simulink model "bustest"  (R2018a)
settings: Solver=VariableStepAuto  StartTime=0.0  StopTime=10.0  RelTol=1e-3
undefined symbols (not defined in the file or in its folder): BaseVoltage, ControlModes, ILDC, m, n, RCReg1, Reg1i, Reg1v, TReg1
(part 1 of 2)
settings Model: Creator=Michael Girbino  LastModifiedBy=Michael Girbino
settings CodeAppCC: StateflowObjectComments=on

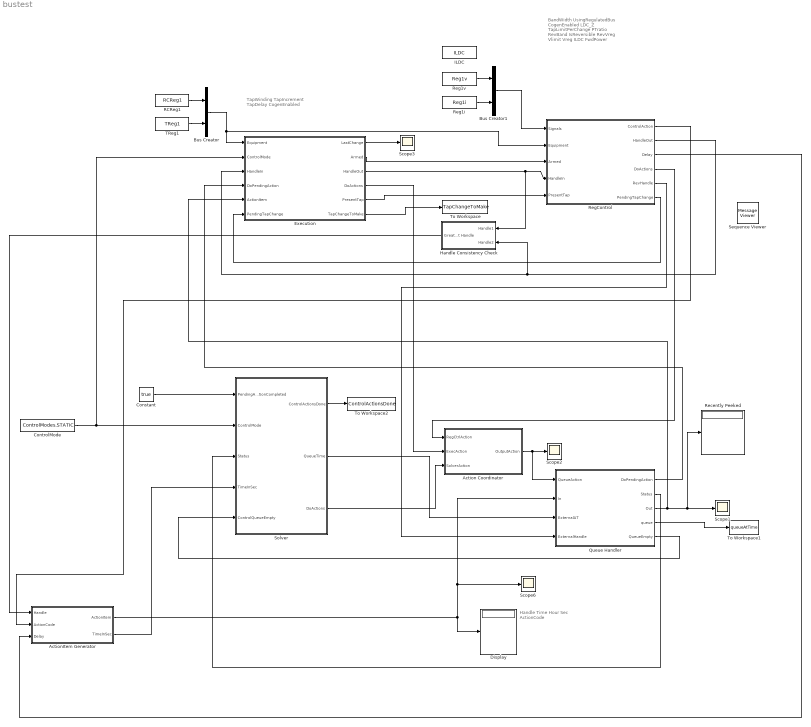
== system bustest ==
  note: BandWidth
      | UsingRegulatedBus
      | CogenEnabled
      | LDC_Z
      | TapLimitPerChange
      | PTratio
      | RevBand
      | IsReversible
      | RevVreg
      | Vlimit
      | Vreg
      | ILDC
      | FwdPower
  note: Handle
      | Time
      | Hour
      | Sec
      | ActionCode
  note: TapWinding
      | TapIncrement
      | TapDelay
      | CogenEnabled
  Action Coordinator : Stateflow chart  TreatAsAtomicUnit=on
  ActionItem Generator : Subsystem
  Bus Creator : BusCreator  Inputs=2  OutDataTypeStr=Bus: EquipmentBus
  Bus Creator1 : BusCreator  Inputs=2  OutDataTypeStr=Bus: SignalBus
  Constant : Constant  Value=true  OutDataTypeStr=boolean
  ControlMode : Constant  Value=ControlModes.STATIC  OutDataTypeStr=Enum: ControlModes
  Display : Display
  Execution : Stateflow chart  TreatAsAtomicUnit=on
  Handle Consistency Check : Subsystem
  ILDC : Constant  Value=ILDC
  Queue Handler : Stateflow chart  TreatAsAtomicUnit=on
  RCReg1 : Constant  Value=RCReg1
  Recently Peeked : Display
  Reg1i : Constant  Value=Reg1i
  Reg1v : Constant  Value=Reg1v
  RegControl : Stateflow chart  TreatAsAtomicUnit=on
  Scope{1..3,6} (4 alike) : Scope
  Sequence Viewer : MessageViewer
  Solver : Stateflow chart  TreatAsAtomicUnit=on
  TReg1 : Constant  Value=TReg1
  To Workspace : ToWorkspace  VariableName=TapChangeToMake  SaveFormat=Timeseries  SampleTime=-1
  To Workspace1 : ToWorkspace  VariableName=queueAtTime  SaveFormat=Structure With Time  SampleTime=-1
  To Workspace2 : ToWorkspace  VariableName=ControlActionsDone  SaveFormat=Timeseries  SampleTime=-1
  wires:
  Queue Handler/5(QueueEmpty) -> Solver/5(ControlQueueEmpty)
  Queue Handler/4(queue) -> To Workspace1/1
  Constant/1 -> Solver/1(PendingActionCompleted)
  ActionItem Generator/2(TimeInSec) -> Solver/4(TimeInSec)
  Queue Handler/2(Status) -> Solver/3(Status)
  ControlMode/1 -> Execution/2(ControlMode), Solver/2(ControlMode)
  Solver/2(QueueTime) -> Queue Handler/3(ExternalAT)
  Queue Handler/3(Out) -> Recently Peeked/1, Scope1/1, Execution/5(ActionItem)
  ActionItem Generator/1(ActionItem) -> Scope6/1, Queue Handler/2(In), Display/1
  Solver/1(ControlActionsDone) -> To Workspace2/1
  RegControl/1(ControlAction) -> ActionItem Generator/2(ActionCode)
  Action Coordinator/1(OutputAction) -> Queue Handler/1(QueueAction), Scope2/1
  Solver/3(DoActions) -> Action Coordinator/3(SolverAction)
  Execution/4(DoActions) -> Action Coordinator/2(ExecAction)
  RegControl/4(DoActions) -> Action Coordinator/1(RegCtrlAction)
  RegControl/3(Delay) -> ActionItem Generator/3(Delay)
  RegControl/2(HandleOut) -> Handle Consistency Check/2(Handle2), Execution/3(HandleIn)
  RegControl/5(RevHandle) -> Queue Handler/4(ExternalHandle)
  Execution/3(HandleOut) -> Handle Consistency Check/1(Handle1), RegControl/4(HandleIn)
  Execution/2(Armed) -> RegControl/3(Armed)
  Queue Handler/1(DoPendingAction) -> Execution/4(DoPendingAction)
  Execution/6(TapChangeToMake) -> To Workspace/1
  RegControl/6(PendingTapChange) -> Execution/6(PendingTapChange)
  Execution/1(LastChange) -> Scope3/1
  Handle Consistency Check/1(Greatest Handle) -> ActionItem Generator/1(Handle)
  Execution/5(PresentTap) -> RegControl/5(PresentTap)
  RCReg1/1 -> Bus Creator/1
  TReg1/1 -> Bus Creator/2
  Reg1v/1 -> Bus Creator1/1
  Reg1i/1 -> Bus Creator1/2
  Bus Creator/1 -> RegControl/2(Equipment), Execution/1(Equipment)
  Bus Creator1/1 -> RegControl/1(Signals)

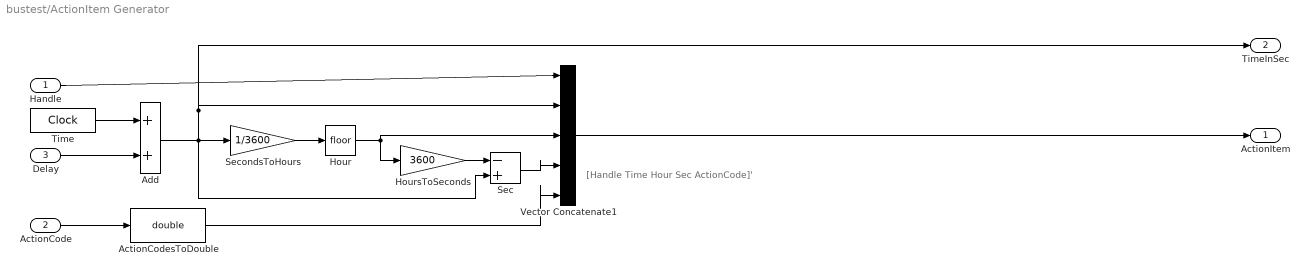
== system bustest/ActionItem Generator ==
  note: [Handle Time Hour Sec ActionCode]'
  Handle : Inport
  ActionCode : Inport  Port=2
  Delay : Inport  Port=3
  ActionCodesToDouble : DataTypeConversion  OutDataTypeStr=double
  Add : Sum
  Hour : Rounding
  HoursToSeconds : Gain  Gain=3600
  Sec : Sum  Inputs=-+
  SecondsToHours : Gain  Gain=1/3600
  Time : DigitalClock
  Vector Concatenate1 : Concatenate  NumInputs=5
  ActionItem : Outport
  TimeInSec : Outport  Port=2
  wires:
  Add/1 -> Sec/2, SecondsToHours/1, TimeInSec/1, Vector Concatenate1/2
  Hour/1 -> Vector Concatenate1/3, HoursToSeconds/1
  SecondsToHours/1 -> Hour/1
  Vector Concatenate1/1 -> ActionItem/1
  HoursToSeconds/1 -> Sec/1
  Handle/1 -> Vector Concatenate1/1
  Sec/1 -> Vector Concatenate1/4
  Delay/1 -> Add/2
  Time/1 -> Add/1
  ActionCode/1 -> ActionCodesToDouble/1
  ActionCodesToDouble/1 -> Vector Concatenate1/5

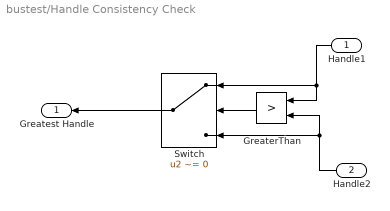
== system bustest/Handle Consistency Check ==
  Handle1 : Inport
  Handle2 : Inport  Port=2
  GreaterThan : RelationalOperator  Operator=>  RndMeth=Simplest
  Switch : Switch  Criteria=u2 ~= 0
  Greatest Handle : Outport
  wires:
  Handle2/1 -> GreaterThan/2, Switch/3
  GreaterThan/1 -> Switch/2
  Handle1/1 -> GreaterThan/1, Switch/1
  Switch/1 -> Greatest Handle/1

== stateflow chart bustest/Execution ==
  settings: executeAtInitialization=1
  state Push(CodeVal, DelayVal) [function]
    (default) -> (junction 341) : {ActionCode = CodeVal;
        | Delay = DelayVal;
        | HandleOut = HandleOut + 1;
        | DoActions.data = QueueActions.PUSH;
        | send(DoActions);}
  state ControlFlow
    state MakingTapChange
      state StaticTapChange
        (default) -> (junction 165) : {TapChangeToMake = AtLeastOneTap(PendingTapChange, TapIncrement(TapWinding));
            | % reset to no change = change - 1 program will determin if another is needed:
            | PendingTapChange = 0;
            | Armed = false;}
      state EventDrivenTapChange
        (default) -> (junction 189) : {[TapChangeToMake LocalPendingTapChange] =...
            |  OneInDirectionOf(LocalPendingTapChange, TapIncrement(TapWinding));
            | PresentTap(TapWinding) = PresentTap(TapWinding) + TapChangeToMake;}
        (junction 189) -> (junction 190) [order 1] : [PendingTapChange ~= 0]
        (junction 189) -> (junction 191) [order 2] : {Armed = false;}
        (junction 190) -> (junction 192) : {Push(ActionCodes.ACTION_TAPCHANGE, TapDelay);}
        (junction 192) -> (junction 191)
      state TimeDrivenTapChange
        (default) -> (junction 200) : {[TapChangeToMake LocalPendingTapChange] =...
            |  OneInDirectionOf(LocalPendingTapChange, TapIncrement(TapWinding));
            | PresentTap(TapWinding) = PresentTap(TapWinding) + TapChangeToMake;}
        (junction 200) -> (junction 202) [order 1] : [PendingTapChange ~= 0]
        (junction 200) -> (junction 203) [order 2] : {Armed = false;}
        (junction 202) -> (junction 201) : {Push(ActionCodes.ACTION_TAPCHANGE, TapDelay);}
        (junction 201) -> (junction 203)
      state MultiRateTapChange
        (default) -> (junction 210) : {[TapChangeToMake, LocalPendingTapChange] =...
            |  OneInDirectionOf(LocalPendingTapChange, TapIncrement(TapWinding));
            | PresentTap(TapWinding) = PresentTap(TapWinding) + TapChangeToMake;}
        (junction 210) -> (junction 212) [order 1] : [PendingTapChange ~= 0]
        (junction 210) -> (junction 213) [order 2] : {Armed = false;}
        (junction 212) -> (junction 211) : {Push(ActionCodes.ACTION_TAPCHANGE, TapDelay);}
        (junction 211) -> (junction 213)
      state Finished
        en: EXIT_TAPCHANGE = true;
      (default) -> (junction 132)
      (junction 132) -> (junction 133) [order 1] : % Check to make sure control has not reset:
          | [PendingTapChange == 0]
      (junction 132) -> (junction 163) [order 2]
      (junction 133) -> (junction 135) : {Armed = false;}
      (junction 163) -> StaticTapChange [order 1] : [ControlMode == ControlModes.STATIC]
      (junction 163) -> (junction 167) [order 2]
      StaticTapChange -> (junction 170)
      (junction 167) -> EventDrivenTapChange [order 1] : [ControlMode == ControlModes.EVENTDRIVEN]
      (junction 167) -> (junction 171) [order 2]
      EventDrivenTapChange -> (junction 169)
      (junction 169) -> (junction 170)
      (junction 170) -> (junction 174)
      (junction 171) -> TimeDrivenTapChange [order 1] : [ControlMode == ControlModes.TIMEDRIVEN]
      (junction 171) -> (junction 175) [order 2]
      TimeDrivenTapChange -> (junction 173)
      (junction 173) -> (junction 174)
      (junction 174) -> (junction 178)
      (junction 175) -> MultiRateTapChange [order 1] : [ControlMode == ControlModes.MULTIRATE]
      (junction 175) -> (junction 179) [order 2]
      (junction 178) -> (junction 180)
      MultiRateTapChange -> (junction 357)
      (junction 357) -> (junction 179)
      (junction 180) -> (junction 357)
      (junction 179) -> ControlFlow.MakingTapChange.Finished
      (junction 135) -> ControlFlow.MakingTapChange.Finished
    state Reversing
      state FlipCogen
        (default) -> (junction 252)
        (junction 252) -> (junction 253) [order 1] : [InCogenMode]
        (junction 252) -> (junction 254) [order 2] : {InCogenMode = true;}
        (junction 253) -> (junction 255) : {InCogenMode = false;}
        (junction 255) -> (junction 254)
      state FlipReverse
        (default) -> (junction 263)
        (junction 263) -> (junction 264) [order 1] : [InReverseMode]
        (junction 263) -> (junction 265) [order 2] : {InReverseMode = true;}
        (junction 264) -> (junction 266) : {InReverseMode = false;}
        (junction 266) -> (junction 265)
      state Finished
        en: EXIT_REVERSE = true;
      (default) -> (junction 229)
      (junction 229) -> (junction 230) [order 1] : [ReversePending]
      (junction 229) -> (junction 231) [order 2]
      (junction 230) -> (junction 242)
      (junction 242) -> (junction 238) [order 1] : [CogenEnabled]
      (junction 242) -> FlipReverse [order 2]
      (junction 238) -> FlipCogen : % Cogen mode takes precedence if present
      FlipCogen -> (junction 245)
      FlipReverse -> (junction 240)
      (junction 245) -> (junction 240)
      (junction 240) -> (junction 232) : {ReversePending = false;}
      (junction 232) -> (junction 231)
      (junction 231) -> ControlFlow.Reversing.Finished
    state Finished
    (default) -> (junction 115) : {AssignInputsToLocals();
        | ResetTransitionFlags();}
    (junction 115) -> MakingTapChange [order 1] : [Code == ActionCodes.ACTION_TAPCHANGE]
    (junction 115) -> (junction 119) [order 2]
    MakingTapChange -> (junction 117) : [EXIT_TAPCHANGE]
    (junction 117) -> (junction 118)
    (junction 118) -> (junction 122)
    (junction 119) -> Reversing [order 1] : [Code == ActionCodes.ACTION_REVERSE]
    (junction 119) -> (junction 123) [order 2]
    Reversing -> (junction 122)
    (junction 122) -> (junction 124) : [EXIT_REVERSE]
    (junction 124) -> (junction 123)
    (junction 123) -> ControlFlow.Finished
  state AssignInputsToLocals [function]
    note: TapWinding
        | TapIncrement
        | TapDelay
        | CogenEnabled
    (default) -> (junction 365) : {% From Script:
        | TapWinding = Equipment.RCReg1.xsfWinding;
        | TapIncrement = Equipment.TReg1.Winding(TapWinding).TapIncrement;
        | TapDelay = Equipment.RCReg1.TapDelay;
        | CogenEnabled = Equipment.RCReg1.CogenEnabled;
        | % From the ControlQueue:
        | Code = ...
        | ActionItem(NewControlQueueFields.ActionCode);
        | % PendingTapChange:
        | LocalPendingTapChange = PendingTapChange;}
    (junction 365) -> (junction 372) [order 1] : [HandleIn > HandleOut]
    (junction 365) -> (junction 373) [order 2]
    (junction 372) -> (junction 374) : {HandleOut = HandleIn;}
    (junction 374) -> (junction 373)
    (junction 373) -> (junction 375)
  state ChangeToMake = AtLeastOneTap(ProposedChange, Increment) [function]
    note: Called in STATIC mode
        | Changes 70% of the way but at least one tap, subject to maximum allowable tap change
    (default) -> (junction 283) : {NumTaps = floor(0.7 * abs(ProposedChange)/Increment);}
    (junction 283) -> (junction 284) [order 1] : [NumTaps == 0]
    (junction 283) -> (junction 285) [order 2]
    (junction 284) -> (junction 286) : {NumTaps = 1;} % At least 1 tap
    (junction 286) -> (junction 285)
    (junction 285) -> (junction 293)
    (junction 293) -> (junction 290) [order 1] : [NumTaps > TapLimitPerChange]
    (junction 293) -> (junction 294) [order 2]
    (junction 290) -> (junction 295) : {NumTaps = TapLimitPerChange;} % Bound by maximum
    (junction 295) -> (junction 294)
    (junction 294) -> (junction 302) : {LastChange = NumTaps;}
    (junction 302) -> (junction 303) [order 1] : % Check sign on change:
        | [ProposedChange > 0]
    (junction 302) -> (junction 304) [order 2] : {ChangeToMake = -1*NumTaps*Increment;
        | LastChange = -1*NumTaps;}
    (junction 303) -> (junction 305) : {ChangeToMake =...
        |  NumTaps*Increment;}
    (junction 305) -> (junction 304)
    (junction 304) -> (junction 306)
  state ResetTransitionFlags [function]
    (default) -> (junction 377) : {EXIT_TAPCHANGE = false;
        | EXIT_REVERSE = false;}
  state [ChangeToMake, NewProposedChange] = OneInDirectionOf(ProposedChange, Increment) [function]
    note: Computes the amount of one tap change in the direction of the pending tapchange
        | Automatically decrements the proposed change by that amount
    (default) -> (junction 318) : {LastChange = 0;}
    (junction 318) -> (junction 319) [order 1] : [ProposedChange > 0]
    (junction 318) -> (junction 320) [order 2] : {ChangeToMake = -1*Increment;
        | LastChange = -1;
        | NewProposedChange = ProposedChange + Increment;}
    (junction 319) -> (junction 321) : {ChangeToMake = Increment;
        | LastChange = 1;
        | NewProposedChange =...
        |  ProposedChange - Increment;}
    (junction 321) -> (junction 320)
    (junction 320) -> (junction 329)
    (junction 329) -> (junction 330) [order 1] : [abs(NewProposedChange) < 0.9*Increment]
    (junction 329) -> (junction 331) [order 2]
    (junction 330) -> (junction 332) : {NewProposedChange = 0;}
    (junction 332) -> (junction 331)
    (junction 331) -> (junction 333)
  (default) -> ControlFlow : DoPendingAction
  data: CodeVal function_input; DelayVal function_input; ProposedChange function_input; Increment function_input; ChangeToMake function_output; ProposedChange function_input; Increment function_input; ChangeToMake function_output; NewProposedChange function_output; Equipment input Bus: EquipmentBus; LastChange output double; Change local double; NumTaps local uint8; ControlMode input Enum: ControlModes; HandleIn input double; Armed output boolean; HandleOut output double =0; DoActions output boolean =false; PresentTap output double; EXIT_REVERSE local boolean; InReverseMode local boolean; EXIT_TAPCHANGE local boolean; ReversePending local boolean; InCogenMode local boolean; DoPendingAction input boolean; TapWinding local uint8; TapIncrement local double; TapDelay local double; CogenEnabled local boolean =false; Code local Enum: ActionCodes; ActionItem input double size=[1 5]; TapChangeToMake output double; PendingTapChange input double; LocalPendingTapChange local double

== stateflow chart bustest/Solver ==
  state ControlFlow
    note: Static
        | - placeholder QueueTime
        | - DoNearestActions
    note: Event-driven
        | - QueueTime is current time
        | - DoNearestActions
    note: Time-driven
        | - QueueTime is current time
        | - DoActions
    note: Multirate
        | - QueueTime is current time
        | - DoMultiRate
    (default) -> (junction 25)
    (junction 25) -> (junction 26) [order 1] : [ControlMode == ControlModes.STATIC]
    (junction 25) -> (junction 29) [order 2]
    (junction 26) -> (junction 54)
    (junction 54) -> (junction 55) [order 1] : [LocalControlQueueEmpty]
        | % execute nearest set of control actions, but leave time where it is
    (junction 54) -> (junction 56) [order 2] : {QueueTime = 0; %[0 0] xHour, xSec
        | DoActions.data = QueueActions.DO_NEAREST_ACTIONS;
        | send(DoActions);
        | % ignores time advancement
        | }
    (junction 55) -> (junction 57) : {ControlActionsDone = true;}
    (junction 57) -> (junction 56)
    (junction 56) -> (junction 27)
    (junction 27) -> (junction 28)
    (junction 28) -> (junction 32)
    (junction 29) -> (junction 30) [order 1] : [ControlMode == ControlModes.EVENTDRIVEN]
        | % execute nearest set of control actions and advance time to that time
    (junction 30) -> (junction 65) : {QueueTime = TimeInSec; %xHour, xSec
        | DoActions.data = QueueActions.DO_NEAREST_ACTIONS;
        | send(DoActions);}
    (junction 29) -> (junction 33) [order 2]
    (junction 65) -> (junction 66) [order 1] : [~PendingActionCompleted]
    (junction 65) -> (junction 67) [order 2]
    (junction 66) -> (junction 68) : {ControlActionsDone = true;
        | % advances time to the next event
        | }
    (junction 68) -> (junction 67)
    (junction 67) -> (junction 31)
    (junction 31) -> (junction 32)
    (junction 32) -> (junction 36)
    (junction 33) -> (junction 34) [order 1] : [ControlMode == ControlModes.TIMEDRIVEN]
        |  % Do all actions having and action time <= specified time
    (junction 33) -> (junction 37) [order 2]
    (junction 34) -> (junction 78) : {QueueTime = TimeInSec; %xHour, xSec
        | DoActions.data = QueueActions.DO_ACTIONS;
        | send(DoActions);}
    (junction 78) -> (junction 80) [order 1] : [~PendingActionCompleted]
    (junction 78) -> (junction 79) [order 2]
    (junction 80) -> (junction 82) : {ControlActionsDone = true;
        | }
    (junction 82) -> (junction 79)
    (junction 79) -> (junction 35)
    (junction 35) -> (junction 36)
    (junction 36) -> (junction 40)
    (junction 37) -> (junction 38) [order 1] : [ControlMode == ControlModes.MULTIRATE]
        |  % Execute the nearest set of control actions, but leave time where it is
    (junction 37) -> (junction 41) [order 2]
    (junction 38) -> (junction 91) : {QueueTime =TimeInSec; %xHour, xSec
        | DoActions.data = QueueActions.DO_MULTIRATE;
        | send(DoActions);}
    (junction 91) -> (junction 88) [order 1] : [~PendingActionCompleted]
    (junction 91) -> (junction 87) [order 2]
    (junction 88) -> (junction 92) : {ControlActionsDone = true;
        | }
    (junction 92) -> (junction 87)
    (junction 87) -> (junction 39)
    (junction 39) -> (junction 40)
    (junction 40) -> (junction 42)
    (junction 42) -> (junction 41)
    (junction 41) -> (junction 43)
  state QueueEmptyCase
    en: LocalControlQueueEmpty = true;
  (default) -> ControlFlow
  QueueEmptyCase -> ControlFlow
  ControlFlow -> QueueEmptyCase : ControlQueueEmpty
  data: ControlActionsDone output boolean; QueueTime output double; DoActions output Enum: QueueActions; PendingActionCompleted input boolean; ControlMode input Enum: ControlModes; ii local double =0; Status input Enum: Statuses; TimeInSec input double; LocalControlQueueEmpty local boolean =false; ControlQueueEmpty input boolean

== stateflow chart bustest/RegControl ==
  settings: executeAtInitialization=1
  state ControlFlow
    state DetermineReversePendingLookingForward
      state CorrectFalseReversePending
        (default) -> (junction 108)
        (junction 108) -> (junction 109) [order 1] : [FwdPower < (-1*RevPowerThreshold)]
        (junction 108) -> (junction 111) [order 2]
        (junction 109) -> (junction 112) : {ReversePending = true;
            | RevHandle = ...
            | Push(ActionCodes.ACTION_REVERSE, ...
            | RevDelay);
            | }
        (junction 112) -> (junction 111)
      state CorrectTrueReversePending
        (default) -> (junction 804)
        (junction 804) -> (junction 123) [order 1] : [FwdPower >= (-1*RevPowerThreshold)]
        (junction 804) -> (junction 809) [order 2]
        (junction 123) -> (junction 806) : % Reset ReversePending:
            | % Delete RevHandle from ControlQueue
            | {DoActions.data = QueueActions.DELETE;
            | send(DoActions);
            | ReversePending = false;
            | RevHandle = 0;}
        (junction 806) -> (junction 809)
      state Finished
        en: GET_VOLTAGE = true;
      (default) -> (junction 106) : {%FwdPower = -1*real( ControlledTransformer.Power(ElementTerminal) );
          | FwdPower = -1*real( ControlledTransformerPower );}
          | % Should we reverse?
      (junction 106) -> ControlFlow.DetermineReversePendingLookingForward.CorrectFalseReversePending [order 1] : [~ReversePending]
      (junction 106) -> (junction 110) [order 2]
      ControlFlow.DetermineReversePendingLookingForward.CorrectFalseReversePending -> (junction 110)
      (junction 110) -> (junction 120)
      (junction 120) -> ControlFlow.DetermineReversePendingLookingForward.CorrectTrueReversePending [order 1] : [ReversePending]
      (junction 120) -> (junction 122) [order 2]
      ControlFlow.DetermineReversePendingLookingForward.CorrectTrueReversePending -> (junction 122)
      (junction 122) -> ControlFlow.DetermineReversePendingLookingForward.Finished
    state DetermineReversePendingLookingReverseOrCogen
      state CorrectFalseReversePending
        (default) -> (junction 130)
        (junction 130) -> (junction 138) [order 1] : [FwdPower > RevPowerThreshold]
        (junction 130) -> (junction 137) [order 2]
        (junction 138) -> (junction 136) : {ReversePending = true;
            | RevHandle = ...
            | Push(ActionCodes.ACTION_REVERSE, ...
            | RevDelay);
            | }
        (junction 136) -> (junction 137)
      state CorrectTrueReversePending
        (default) -> (junction 154)
        (junction 154) -> (junction 799) [order 1] : [FwdPower <= RevPowerThreshold]
        (junction 154) -> (junction 792) [order 2]
        (junction 799) -> (junction 148) : % Reset ReversePending:
            | {ReversePending = false;}
        (junction 148) -> (junction 792)
      state Finished
        en: REV_NEUTRAL = true;
      (default) -> (junction 144) : {%%FwdPower = -1*real( ControlledTransformer.Power(ElementTerminal) );
          | FwdPower = -1*real( ControlledTransformerPower );}
          | % If reversed, check if power is back in forward direction
      (junction 144) -> ControlFlow.DetermineReversePendingLookingReverseOrCogen.CorrectFalseReversePending [order 1] : [~ReversePending]
      (junction 144) -> (junction 139) [order 2]
      ControlFlow.DetermineReversePendingLookingReverseOrCogen.CorrectFalseReversePending -> (junction 139)
      (junction 139) -> (junction 147)
      (junction 147) -> ControlFlow.DetermineReversePendingLookingReverseOrCogen.CorrectTrueReversePending [order 1] : [ReversePending]
      (junction 147) -> (junction 151) [order 2]
      ControlFlow.DetermineReversePendingLookingReverseOrCogen.CorrectTrueReversePending -> (junction 151)
      (junction 151) -> ControlFlow.DetermineReversePendingLookingReverseOrCogen.Finished
    state ReverseNeutralCase
      state Finished
        send(GET_VOLTAGE);
      state Exiting
        en: EXIT = true;
      (default) -> (junction 166)
      (junction 166) -> (junction 155) [order 1] : % tap change not specified as needed:
          | [~Armed]
      (junction 166) -> ControlFlow.ReverseNeutralCase.Finished [order 2]
      (junction 155) -> (junction 160) : {PendingTapChange = 0.0;}
      (junction 160) -> (junction 167) [order 1] : [abs(PresentTap(TapWinding) - 1.0) < EPSILON]
      (junction 160) -> Exiting [order 2]
      (junction 167) -> (junction 518) : {Increment = TapIncrement(TapWinding);
          | PendingTapChange = round( (1.0 - ...
          | PresentTap(TapWinding)) / Increment ) * Increment;}
      (junction 518) -> (junction 519) [order 1] : [PendingTapChange ~= 0.0 && ~Armed]
      (junction 519) -> (junction 521) : {% Push ACTION_TAPCHANGE
          | % to ControlQueue with TapDelay:
          | Push(ActionCodes.ACTION_TAPCHANGE, TapDelay);
          | Armed = true;}
      (junction 518) -> (junction 520) [order 2]
      (junction 521) -> (junction 520)
      (junction 520) -> (junction 164)
      (junction 164) -> Exiting
    state GetVoltage
      state Finished
        en: DETERMINE_VLOCALBUS = true;
      (default) -> (junction 75)
      (junction 75) -> (junction 76) [order 1] : [UsingRegulatedBus]
      (junction 75) -> ControlFlow.GetVoltage.Finished [order 2] : {VBuffer = ControlledTransformerWindingVoltages;
          | %ControlledTransformer.GetWindingVoltages;
          | Vcontrol = GetControlVoltage;}
      (junction 76) -> (junction 78) : {TransformerConnection = ControlledTransformerConnection;
          | %TransformerConnection = ControlledTransformer.Winding(ElementTerminal).Connection;
          | Vterminal = ComputeVTerminal;}
      (junction 78) -> ControlFlow.GetVoltage.Finished
    state DetermineVlocalbus
      state Finished
        en: GET_VOLTAGEWLDC = true;
      (default) -> (junction 321)
      (junction 321) -> (junction 322) [order 1] : % Voltage limit for bus connected to regulated winding; default = 0.0 (inactive)
          | [VlimitActive]
      (junction 321) -> ControlFlow.DetermineVlocalbus.Finished [order 2] : {Vlocalbus = 0.0;}
      (junction 322) -> (junction 332)
      (junction 332) -> (junction 333) [order 1] : % when controlled transformer is different from LDC PTransformer
          | [UsingRegulatedBus]
      (junction 332) -> (junction 334) [order 2] : % controlled transformer is
          | % the LDC PTransformer
          | {Vlocalbus = abs(Vcontrol);}
      (junction 333) -> (junction 335) : {%ControlledTransformer.GetWindingVoltages(ElementTerminal, VBuffer);
          | Vlocalbus = abs( VBuffer(1) / PTRatio );}
      (junction 335) -> (junction 334)
      (junction 334) -> (junction 324)
      (junction 324) -> ControlFlow.DetermineVlocalbus.Finished
    state GetVoltageWithLDC
      state RX_LDCmode
        (default) -> (junction 365)
        (junction 365) -> (junction 366) [order 1] : [InReverseMode || InCogenMode]
        (junction 365) -> (junction 367) [order 2] : {VLDC = complex(R, X) * complex( real(ILDC), imag(ILDC) );}
        (junction 366) -> (junction 368) : {VLDC = complex(revR, revX) * complex( real(ILDC), imag(ILDC) );}
        (junction 368) -> (junction 367)
      state Z_LDCmode
        (default) -> (junction 387)
        (junction 387) -> (junction 388) [order 1] : [InReverseMode || InCogenMode]
        (junction 387) -> (junction 389) [order 2] : {Vcontrol = abs(Vcontrol) - abs(ILDC) * LDC_Z;}
        (junction 388) -> (junction 390) : {Vcontrol = abs(Vcontrol) - abs(ILDC) * revLDC_Z;}
        (junction 390) -> (junction 389)
      state Finished
        en: GET_TEST_VALUES = true;
      (default) -> (junction 354) : {%%ControlledElement.GetCurrents(CBuffer);
          | %Convert current to control current by CTRating:
          | ILDC = ControlledElementCurrents( ControlledElementNconds * (ElementTerminal - 1) + ControlledPhase);}
      (junction 354) -> RX_LDCmode [order 1] : % Standard R, X LDC
          | [LDC_Z == 0.0]
      (junction 354) -> Z_LDCmode [order 2] : % Beckwith LDC_Z control mode
      Z_LDCmode -> ControlFlow.GetVoltageWithLDC.Finished
      RX_LDCmode -> ControlFlow.GetVoltageWithLDC.Finished
    state GetTestValues
      state Finished
        en:
        DETERMINE_TAP_CHANGE = true;
      (default) -> (junction 398) : % assumes looking forward:
          | {Vactual = abs(Vcontrol);}
      (junction 398) -> (junction 399) [order 1] : [InReverseMode]
      (junction 398) -> ControlFlow.GetTestValues.Finished [order 2] : {VregTest = Vreg;
          | BandTest = Bandwidth;}
      (junction 399) -> (junction 401) : {Vactual = Vactual / PresentTap(TapWinding);
          | VregTest = RevVreg;
          | BandTest = RevBandwidth;}
      (junction 401) -> ControlFlow.GetTestValues.Finished
    state DetermineTapChangeIsNeeded
      state Finished
        en:
        MAKE_TAP_CHANGE = true;
      (default) -> (junction 409)
      (junction 409) -> (junction 410) [order 1] : % difference between desired and actual > half bandwidth
          | [abs(VregTest - Vactual) > BandTest/2.0]
      (junction 409) -> ControlFlow.DetermineTapChangeIsNeeded.Finished [order 2] : {TapChangeIsNeeded = false;}
      (junction 410) -> (junction 412) : {TapChangeIsNeeded = true;}
      (junction 412) -> ControlFlow.DetermineTapChangeIsNeeded.Finished
    state MakeTapChange
      state GetVboostFromVlimit
        (default) -> (junction 441)
        (junction 441) -> (junction 446) [order 1] : [Vlocalbus > Vlimit]
        (junction 441) -> (junction 443) [order 2]
        (junction 446) -> (junction 445) : {Vboost = Vlimit - Vlocalbus;}
        (junction 445) -> (junction 443)
      state TapChangeUp
        (default) -> (junction 475)
        (junction 475) -> (junction 476) [order 1] : [PresentTap(TapWinding) < MaxTap(TapWinding)]
        (junction 475) -> (junction 477) [order 2]
        (junction 476) -> (junction 478) : {% push ACTION_TAPCHANGE to ControlQueue
            | % with delay ComputeTimeDelay(Vactual):
            | Push(ActionCodes.ACTION_TAPCHANGE, ...
            | ComputeTimeDelay(Vactual));
            | Armed = true;}
        (junction 478) -> (junction 477)
      state TapChangeDown
        (default) -> (junction 488) : % going down:
        (junction 488) -> (junction 489) [order 1] : [PresentTap(TapWinding) > MinTap(TapWinding)]
        (junction 488) -> (junction 490) [order 2]
        (junction 489) -> (junction 491) : {% push ACTION_TAPCHANGE to ControlQueue
            | % with delay ComputeTimeDelay(Vactual):
            | Push(ActionCodes.ACTION_TAPCHANGE, ...
            | ComputeTimeDelay(Vactual));
            | Armed = true;}
        (junction 491) -> (junction 490)
      state Finished
        en: FINISHED = true;
      (default) -> (junction 431) : % compute tapchange:
          | {Vboost = VregTest - Vactual;}
      (junction 431) -> (junction 432) [order 1] : [VlimitActive]
      (junction 431) -> (junction 433) [order 2]
      (junction 432) -> GetVboostFromVlimit
      GetVboostFromVlimit -> (junction 434)
      (junction 434) -> (junction 433)
      (junction 433) -> (junction 435) : {% PU winding boost needed:
          | BoostNeeded = Vboost * PTRatio / BaseVoltage(ElementTerminal);
          | Increment = TapIncrement(TapWinding);
          | % quantize to an increment:
          | PendingTapChange = round(BoostNeeded/Increment)*Increment;}
      (junction 435) -> (junction 453) : % send initial tap change message to ControlQueue, add delay time to solution control queue:
      (junction 453) -> (junction 454) [order 1] : % only changes 1 tap at a time:
          | [PendingTapChange ~= 0.0 && ~Armed]
      (junction 453) -> ControlFlow.MakeTapChange.Finished [order 2]
      (junction 454) -> (junction 464) : % see of any tap change is possible in desired direction (not saturated):
      (junction 464) -> TapChangeUp [order 1] : % going up:
          | [PendingTapChange > 0.0]
      (junction 464) -> TapChangeDown [order 2]
      TapChangeUp -> (junction 467)
      TapChangeDown -> (junction 466)
      (junction 467) -> (junction 466)
      (junction 466) -> (junction 456)
      (junction 456) -> ControlFlow.MakeTapChange.Finished
    state Finished
    (default) -> (junction 207) : {AssignInputsToLocals();
        | ResetTransitionFlags();}
    (junction 207) -> (junction 208) [order 2]
    (junction 208) -> (junction 86)
    (junction 207) -> (junction 529) [order 1] : [TapLimitPerChange == 0]
    (junction 86) -> (junction 87) [order 1] : [~UsingRegulatedBus]
    (junction 87) -> (junction 61)
    (junction 86) -> (junction 88) [order 2]
    (junction 61) -> (junction 62) [order 1] : [IsReversible || CogenEnabled]
    (junction 61) -> (junction 65) [order 2]
    (junction 62) -> (junction 63)
    (junction 63) -> DetermineReversePendingLookingForward [order 1] : [LookingForward && ~InCogenMode]
    (junction 63) -> DetermineReversePendingLookingReverseOrCogen [order 2]
    DetermineReversePendingLookingForward -> (junction 67) : [GET_VOLTAGE]
    DetermineReversePendingLookingReverseOrCogen -> (junction 175) : [REV_NEUTRAL]
    (junction 175) -> ReverseNeutralCase [order 1] : % mode for which tap change may be executed,
        | % but no reversal made:
        | [ReverseNeutral]
    (junction 175) -> (junction 174) [order 2]
    ReverseNeutralCase -> (junction 174) [order 2] : GET_VOLTAGE
    (junction 174) -> (junction 127)
    ReverseNeutralCase -> (junction 532) [order 1] : [EXIT]
    (junction 65) -> (junction 88)
    (junction 127) -> (junction 65)
    (junction 67) -> (junction 127)
    (junction 88) -> GetVoltage
    (junction 532) -> (junction 529)
    (junction 529) -> (junction 212)
    GetVoltage -> DetermineVlocalbus : [DETERMINE_VLOCALBUS]
    DetermineVlocalbus -> (junction 343) : [GET_VOLTAGEWLDC]
    (junction 343) -> GetVoltageWithLDC [order 1] : % line drop compensation, but not using regulated bus
        | [~UsingRegulatedBus && LDCActive]
    (junction 343) -> (junction 345) [order 2]
    GetVoltageWithLDC -> (junction 346) : [GET_TEST_VALUES]
    (junction 346) -> (junction 345)
    (junction 345) -> GetTestValues
    GetTestValues -> DetermineTapChangeIsNeeded : [DETERMINE_TAP_CHANGE]
    DetermineTapChangeIsNeeded -> (junction 420) : [MAKE_TAP_CHANGE]
    (junction 420) -> MakeTapChange [order 1] : [TapChangeIsNeeded]
    (junction 420) -> (junction 422) [order 2]
    MakeTapChange -> (junction 423) : [FINISHED]
    (junction 423) -> (junction 422)
    (junction 422) -> ControlFlow.Finished
    (junction 212) -> ControlFlow.Finished : {PendingTapChange = 0;}
  state h = Push(CodeVal, DelayVal) [function]
    (default) -> (junction 860) : {ActionCode = CodeVal;
        | Delay = DelayVal;
        | HandleOut = HandleOut + 1;
        | DoActions.data = QueueActions.PUSH;
        | send(DoActions);
        | h = HandleOut;}
  state AssignInputsToLocals [function]
    (default) -> (junction 987) : {BandWidth = Equipment.RCReg1.Bandwidth;
        | UsingRegulatedBus = Equipment.RCReg1.UsingRegulatedBus;
        | CogenEnabled = Equipment.RCReg1.CogenEnabled;
        | LDC_Z = Equipment.RCReg1.LDC_Z;
        | TapLimitPerChange = Equipment.RCReg1.TapLimitPerChange;
        | PTratio = Equipment.RCReg1.PTRatio;
        | RevBand = Equipment.RCReg1.revBandwidth;
        | RevDelay = Equipment.RCReg1.RevDelay;
        | IsReversible = Equipment.RCReg1.IsReversible;
        | RevVreg = Equipment.RCReg1.RevVreg;
        | RevPowerThreshold = Equipment.RCReg1.revPowerThreshold;
        | Vlimit = Equipment.RCReg1.Vlimit;
        | Vreg = Equipment.RCReg1.Vreg;
        |
        | ILDC = Inputs.ILDC;
        |
        | FwdPower = Signals.Reg1i * Signals.Reg1v;
        | ControlledTransformerPower = ...
        | Signals.Reg1i * Signals.Reg1v;
        | ControlledTransformerWindingVoltages = ...
        | Signals.Reg1v;
        |
        | TapDelay = Equipment.RCReg1.TapDelay;}
    (junction 987) -> (junction 996) [order 1] : [Equipment.RCReg1.R~=0 || Equipment.RCReg1.X~=0 || Equipment.RCReg1.LDC_Z>0]
    (junction 987) -> (junction 991) [order 2] : {LDCActive = false;}
    (junction 996) -> (junction 990) : {LDCActive = true;}
    (junction 990) -> (junction 991)
    (junction 991) -> (junction 722)
    (junction 722) -> (junction 897) [order 1] : [HandleIn > HandleOut]
    (junction 722) -> (junction 898) [order 2]
    (junction 897) -> (junction 899) : {HandleOut = HandleIn;}
    (junction 899) -> (junction 898)
    (junction 898) -> (junction 900)
  note: BandWidth
      | UsingRegulatedBus
      | CogenEnabled
      | LDC_Z
      | TapLimitPerChange
      | PTratio
      | RevBand
      | IsReversible
      | RevVreg
      | Vlimit
      | Vreg
      | ILDC
      | FwdPower
  state ResetTransitionFlags [function]
    (default) -> (junction 886) : {DETERMINE_TAP_CHANGE = false;
        | DETERMINE_VLOCALBUS = false;
        | EXIT = false;
        | FINISHED = false;
        | GET_TEST_VALUES = false;
        | GET_VOLTAGE = false;
        | GET_VOLTAGEWLDC = false;
        | MAKE_TAP_CHANGE = false;
        | REV_NEUTRAL = false;}
  state UpdateControlledTransformerWV [function]
    note: Retrieves new value for ControlledTransformerWindingVoltages. Update since last call of AssignInputsToLocals. Necessary because the control flow requires multiple updates to this quantity.
    (default) -> (junction 905) : {ControlledTransformerWindingVoltages = ...
        | Inputs.ControlledTransformerWindingVoltages;}
  state UpdateControlledTransformerPower [function]
    note: Retrieves new value for ControlledTransformerPower. Update since last call of AssignInputsToLocals. Necessary because the control flow requires multiple updates to this quantity.
    (default) -> (junction 902) : {ControlledTransformerPower = ...
        | Inputs.ControlledTransformerPower;}
  state vt = ComputeVTerminal [function]
    (default) -> (junction 309) : % Iteration through order of admittance matrix
        | % (inherited from CktElement)
    (junction 310) -> (junction 308) [order 1] : [ii <= Yorder]
    (junction 308) -> (junction 311) : {vt(ii) = NodeV(NodeRef(ii));}
    (junction 309) -> (junction 310) : {ii = 1;}
    (junction 311) -> (junction 310) : {ii = ii + 1;}
    (junction 310) -> (junction 312) [order 2]
  state WindingVoltages = GetWindingVoltages(Transformer, IndicatedWinding) [function]
    note: Intend to store WindingVoltages in VBuffer.
        | Fills array with voltages across indicated winding
    note: For Delta connections or Line-Line voltages
    (default) -> (junction 969) : % Determine whether winding exists
    (junction 923) -> (junction 921) [order 1] : [ii <= Yorder]
    (junction 921) -> (junction 924) : {Vterminal(ii) = NodeV( NodeRef(i) );}
    (junction 969) -> (junction 922) [order 1] : [IndicatedWinding >= 1 && IndicatedWinding <= NumWindings]
    (junction 969) -> (junction 971) [order 2]
    (junction 922) -> (junction 923) : {ii = 1;}
    (junction 924) -> (junction 923) : {ii = ii + 1;}
    (junction 923) -> (junction 925) [order 2] : {k = (IndicatedWinding - 1) * Fnconds;
        | NeutTerm = Fnphases + k + 1;}
    (junction 925) -> (junction 935) : {ii = 1;}
    (junction 935) -> (junction 933) [order 1] : [ii <= Fnphases]
    (junction 933) -> (junction 952)
    (junction 952) -> (junction 953) [order 1] : [Winding(IndicatedWinding).Connection == Connections.WYE]
    (junction 952) -> (junction 956) [order 2]
    (junction 953) -> (junction 954) : {VBuffer(ii) = Vterminal(ii + k) - Vterminal(NeutTerm);}
    (junction 954) -> (junction 955)
    (junction 955) -> (junction 959)
    (junction 956) -> (junction 957) [order 1] : [Winding(IndicatedWinding).Connection == Connections.DELTA]
    (junction 956) -> (junction 960) [order 2]
    (junction 957) -> (junction 958) : {iii = RotatePhases(ii);
        | VBuffer(ii) = ...
        | Vterminal(ii + k) - ...
        | Vterminal(iii+k);}
    (junction 936) -> (junction 935) : {ii = ii + 1;}
    (junction 935) -> (junction 937) [order 2] : {WindingVoltages = VBuffer;}
    (junction 958) -> (junction 959)
    (junction 959) -> (junction 961)
    (junction 961) -> (junction 960)
    (junction 960) -> (junction 936)
    (junction 937) -> (junction 971)
    (junction 971) -> (junction 973)
  state Result = GetControlVoltage [function]
    (default) -> (junction 236)
    (junction 236) -> (junction 237) [order 1] : [FPTphase == FPTphases.MAXPHASE]
        | % controlled phase is that with greatest |V|
    (junction 236) -> (junction 240) [order 2]
    (junction 237) -> (junction 260) : {ControlledPhase = 1;
        | % abs is equivalent to Cabs:
        | V = abs( VBuffer(ControlledPhase) );}
        | % Iteration through remaining phases:
    (junction 261) -> (junction 259) [order 1] : [ii <= Nphs]
    (junction 259) -> (junction 270)
    (junction 260) -> (junction 261) : {ii = 2;}
    (junction 270) -> (junction 271) [order 1] : [abs( VBuffer(ControlledPhase)) > V]
        | % if it's GREATER, make it the new V
    (junction 270) -> (junction 272) [order 2]
    (junction 271) -> (junction 273) : {V = VBuffer(ControlledPhase);
        | ControlledPhase = ii;}
    (junction 262) -> (junction 261) : {ii = ii+1;}
    (junction 261) -> (junction 238) [order 2]
    (junction 273) -> (junction 272)
    (junction 272) -> (junction 262) : {Result = VBuffer(FPTphase) / PTRatio;
        | % Complex divided by real
        | }
    (junction 238) -> (junction 239)
    (junction 239) -> (junction 243)
    (junction 240) -> (junction 241) [order 1] : [FPTphase == FPTphases.MINPHASE]
        | % controlled phase is that with least |V|
    (junction 241) -> (junction 282) : {ControlledPhase = 1;
        | % abs is equivalent to Cabs:
        | V = abs( VBuffer(ControlledPhase) );}
        | % Iteration through remaining phases:
    (junction 240) -> (junction 244) [order 2] : % just use one phase because
        | % that's what most controls do:
        | {Result = VBuffer(ControlledPhase) / PTRatio;
        | ControlledPhase = FPTphase;}
    (junction 278) -> (junction 277) [order 1] : [ii <= Nphs]
    (junction 277) -> (junction 291)
    (junction 282) -> (junction 278) : {ii = 2;}
    (junction 291) -> (junction 292) [order 1] : [abs( VBuffer(ControlledPhase)) < V]
        | % if it's LESS, make it the new V
    (junction 291) -> (junction 293) [order 2]
    (junction 292) -> (junction 294) : {V = VBuffer(ControlledPhase);
        | ControlledPhase = ii;}
    (junction 280) -> (junction 278) : {ii = ii+1;}
    (junction 278) -> (junction 242) [order 2]
    (junction 294) -> (junction 293)
    (junction 293) -> (junction 280) : {Result = VBuffer(FPTphase) / PTRatio;
        | % Complex divided by real
        | }
    (junction 242) -> (junction 243)
    (junction 243) -> (junction 245)
    (junction 245) -> (junction 244)
    (junction 244) -> (junction 246)
  state Result = ComputeTimeDelay(Vavg) [function]
    (default) -> (junction 507)
    (junction 507) -> (junction 508) [order 1] : [Finversetime]
    (junction 507) -> (junction 509) [order 2] : % determines which regulator control will act first,
        | % default is 15s
        | {Result = TimeDelay;}
    (junction 508) -> (junction 510) : % TimeDelay is adjusted inversely proportional to
        | % the amount that voltage is outside the band,
        | % down to 10 percent of specified time delay
        | % (Further out of band = band - 1> less time delay)
        | {Result = TimeDelay / min(10.0, 2.0*abs(Vreg - Vavg)/Bandwidth);}
    (junction 510) -> (junction 509)
    (junction 509) -> (junction 511)
  (default) -> ControlFlow
  data: CodeVal function_input; DelayVal function_input; h function_output; vt function_output; IndicatedPhase function_input; RotatedPhase function_output; Transformer function_input; IndicatedWinding function_input; WindingVoltages function_output; Result function_output; Vavg function_input; Result function_output; Signals input Bus: SignalBus; Equipment input Bus: EquipmentBus; BandTest local double =0; BoostNeeded local double =0; Increment local double =0; ReversePending local boolean =false; TapChangeIsNeeded local boolean =false; Vactual local double =0; Vboost local double =0; Vcontrol local double =0; Vlocalbus local double =0; VregTest local double =0; EPSILON local double =1.0e-12; R local double =0; X local double =0; BaseVoltage local double; ControlledPhase local uint8; ElementTerminal local uint8 =1; InCogenMode local boolean =false; InReverseMode local boolean =false; LDCActive local boolean =false; LookingForward local boolean =false; MaxTap local uint8; MinTap local uint8; NodeV local double; RevPowerThreshold local double; ReverseNeutral local boolean =false; TapIncrement local double; TapWinding local uint8 =1; VBuffer local double; VlimitActive local boolean =false; revLDC_Z local double =0; revR local double =0; revX local double =0; TransformerConnection local int32 =0; VLDC local double =0; Vterminal local double; Bandwidth local double =3; CogenEnabled local boolean =false; FwdPower local double =0; ILDC local double =0; IsReversible local boolean =false; LDC_Z local double =0; PTRatio local double =60; RevBandwidth local double =3; RevVreg local double =120; TapLimitPerChange local uint8 =16; UsingRegulatedBus local boolean =false; Vlimit local double =0; Vreg local double =120; ControlAction output Enum: ActionCodes; Armed input boolean =false; HandleOut output double =0; Delay output double =0; DoActions output Enum: QueueActions; RevBackHandle local uint8 =0; RevHandle output uint8 =0; REV_NEUTRAL local boolean =false; RevDelay local double; ControlledTransformerWindingVoltages local double; ControlledTransformerConnection local Enum: Connections; EXIT local boolean =false; FINISHED local boolean =false; GET_TEST_VALUES local boolean =false; MAKE_TAP_CHANGE local boolean =false; DETERMINE_TAP_CHANGE local boolean =false; GET_VOLTAGE local boolean =false; GET_VOLTAGEWLDC local boolean =false; DETERMINE_VLOCALBUS local boolean =false; TapDelay local double; HandleIn input double; PendingTapChange output double; PresentTap input double; ControlledElementCurrents local double; ControlledElementNconds local double; ControlledTransformerPower local double
  function RotatedPhase = RotatePhases(IndicatedPhase):
    | function RotatedPhase = RotatePhases(IndicatedPhase)
    |     HVLeadsLV = false;
    |     % FIRST NEED TO DETERMINE DELTADIRECTION:
    |     % If high voltage is delta, delta leads y (1)
    |     % If high voltage is wye, delta lags wye (2)
    |     if Winding(1).connection = Winding(2).connection
    |         DeltaDirection = 1;
    |     else
    |         if Winding(1).kvll >= Winding(2).kvll
    |             iHvolt = 1;
    |         else
    |             iHVolt = 2;
    |         end
    |         switch Winding(iHvolt).Connection
    |             case 0
    |                 if HVLeadsLV
    |                     DeltaDirection = -1;
    |                 else
    |                     DeltaDirection = 1;
    |                 end
    |             case 1
    |                 if HVLeadsLV
    |                     DeltaDirection = 1;
    |                 else
    |                     DeltaDirection = -1;
    |                 end
    |         end
    |     end
    |     
    |     % NOW, ACTUALLY DETERMINE PHASE ROTATION
    |     RotatedPhase = IndicatedPhase + DeltaDirection;
    | 
    |     % make sure RotatedPhase is within limits:
    |     if fNphases > 2
    |         % Assumes 2 phase delta is open delta
    |         if RotatedPhase > fNphases
    |             RotatedPhase = 1;
    |         elseif RotatedPhase < 1
    |             RotatedPhase = fNphases;
    |         end
    |     elseif RotatedPhase < 1
    |         RotatedPhase = 3; % For 2-phase delta, next phase will be 3rd phase
    |     end
    | end
